simulink model "simulink_"  (R2021b)
settings: Solver=VariableStepAuto  StartTime=0.0  StopTime=10.0  RelTol=1e-3
values from neighbouring files (symbols this model uses):
  A = [0 1; -10^4 -10]    [script.m]
  B = [0; 10^4]    [script.m]
  C = [1 1]    [script.m]
  x0 = [1; 5]    [script.m]
settings Model: Creator=55189  LastModifiedBy=55189

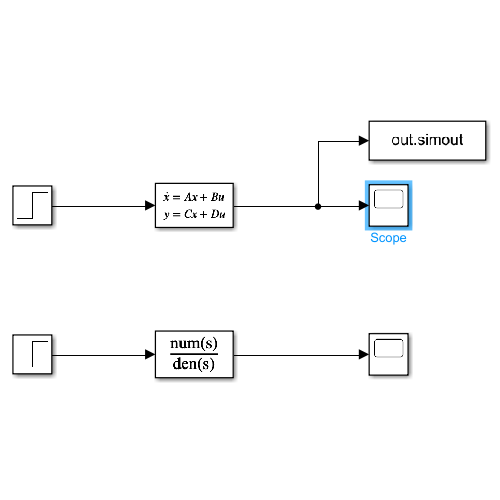
[thumbnail: Simulink's stored preview of the top-level diagram]
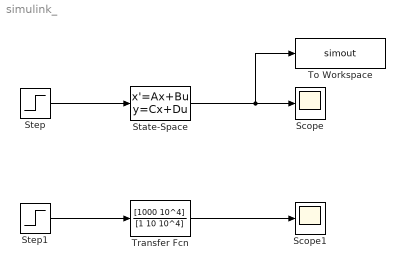
== system simulink_ ==
  Scope : Scope
  Scope1 : Scope
  State-Space : StateSpace  A=A  B=B  C=C  D=[0]  InitialCondition=x0
  Step : Step  Time=0  SampleTime=0
  Step1 : Step  Time=0  SampleTime=0
  To Workspace : ToWorkspace  VariableName=simout  SampleTime=-1
  Transfer Fcn : TransferFcn  Numerator=[1000 10^4]  Denominator=[1 10 10^4]
  wires:
  Step/1 -> State-Space/1
  State-Space/1 -> To Workspace/1, Scope/1
  Transfer Fcn/1 -> Scope1/1
  Step1/1 -> Transfer Fcn/1
